simulink model "FUNCIIONA"  (Simulink 8.4)
settings: Solver=ode45  StartTime=0.0  StopTime=100  RelTol=1e-3
settings Model: Creator=juan  LastModifiedBy=Permuta  ExtModeAutoUpdateStatusClock=off
settings OptimizationCC: ExpressionDepthLimit=128  InitFltsAndDblsToZero=on
settings DebuggingCC: SaveWithParameterizedLinksMsg=none  SignalResolutionControl=TryResolveAllWithWarning  StateNameClashWarn=none
settings GRTTargetCC: TargetFcnLib=ansi_tfl_tmw.mat

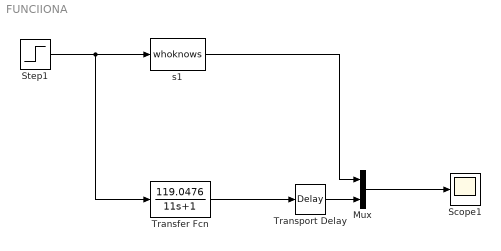
== system FUNCIIONA ==
  Mux : Mux  Inputs=2
  Scope1 : Scope
      settings: SaveName=Parte2
  Step1 : Step  SampleTime=0
  Transfer Fcn : TransferFcn  Numerator=[119.0476]  Denominator=[11 1]
  Transport Delay : TransportDelay  DelayTime=6
  s1 : M-S-Function  FunctionName=whoknows  Parameters=L, P1, P2, T, R  mask{L=7, P1=0, P2=2, T=1, R=0}
      mask prompts: L "Laboratorio"; P1 "Primer digito del Puesto"; P2 "Segundo digito del Puesto"; T "Tipo de Planta"; R "Ruido"
      mask Display: disp('Sistema')
  wires:
  Step1/1 -> Transfer Fcn/1, s1/1
  s1/1 -> Mux/1
  Transfer Fcn/1 -> Transport Delay/1
  Transport Delay/1 -> Mux/2
  Mux/1 -> Scope1/1
